simulink model "Telescope_model_MPC"  (R2024b)
settings: Solver=ode4  StartTime=0.0  StopTime=SimulationTime  FixedStep=Tc  RelTol=1e-5
undefined symbols (not defined in the file): APaz, APel, Arcs2Deg, BPaz, BPel, CPaz, CPel, Deg2Arcs, DPaz, DPel, Prepocessor, Scenario, sgn, VonKarman, x0_az, x0_el
libraries: simulink x18, mpclib x1
(part 1 of 2)
settings Model: Creator=giaco  LastModifiedBy=giacomobasile
settings DebuggingCC: UnderSpecifiedDimensionMsg=warning
settings RTWCC: GPUComputeCapability=3.5

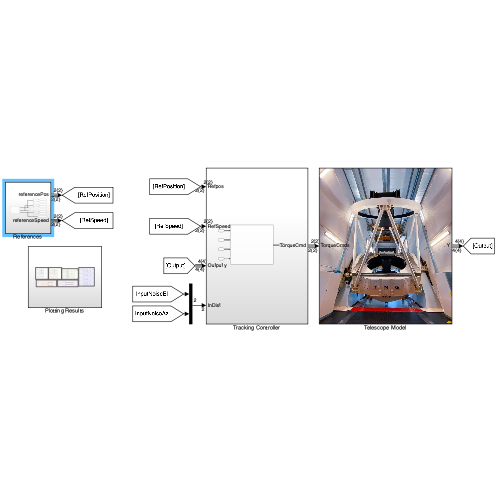
[thumbnail: Simulink's stored preview of the top-level diagram]
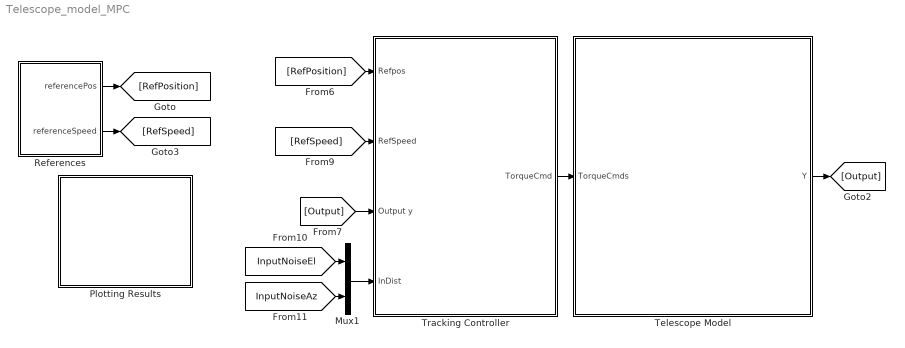
== system Telescope_model_MPC ==
  Mux1 : Mux  Inputs=2
  Plotting Results : Subsystem
  References : Subsystem
  Telescope Model : Subsystem
      mask Display: image('tng1_1.jpg');
  Tracking Controller : Subsystem
  wires:
  [InputNoiseAz] -> Mux1/2
  [RefSpeed] -> Tracking Controller/2(RefSpeed)
  [Output] -> Tracking Controller/3(Output y)
  Mux1/1 -> Tracking Controller/4(InDist)
  [RefPosition] -> Tracking Controller/1(Refpos)
  [InputNoiseEl] -> Mux1/1
  References/2(referenceSpeed) -> [RefSpeed]
  References/1(referencePos) -> [RefPosition]
  Telescope Model/1(Y) -> [Output]
  Tracking Controller/1(TorqueCmd) -> Telescope Model/1(TorqueCmds)

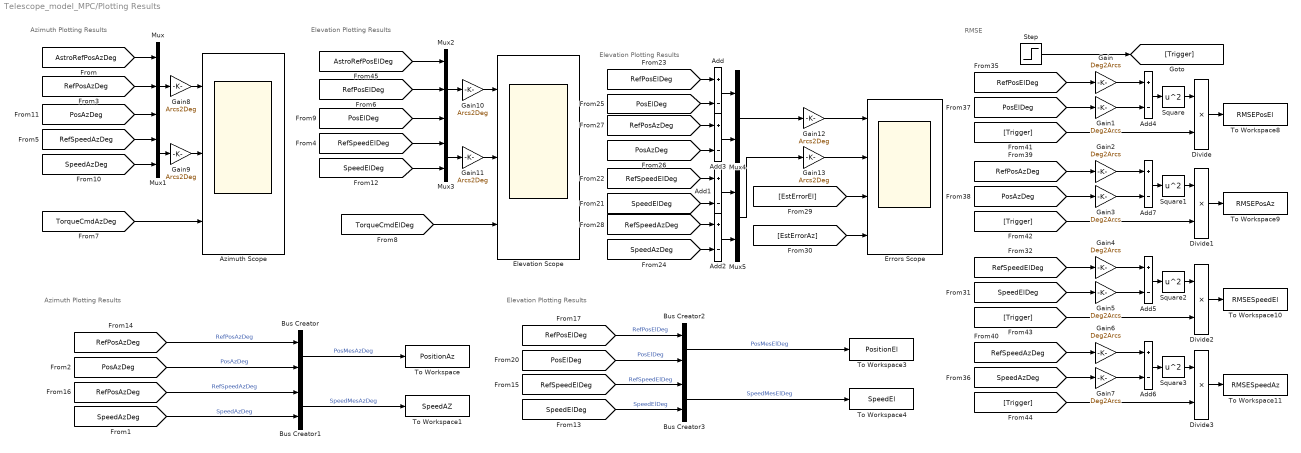
== system Telescope_model_MPC/Plotting Results ==
  note: RMSE
  note: Azimuth Plotting Results
  note: Elevation Plotting Results
  note: Elevation Plotting Results
  note: Azimuth Plotting Results
  note: Elevation Plotting Results
  Add{,1..7} (8 alike) : Sum  Inputs=+-
  Azimuth Scope : Scope  NumInputPorts=3
  Bus Creator{,1..3} (4 alike) : BusCreator  Inputs=2
  Divide{,1..3} (4 alike) : Product  Inputs=**
  Elevation Scope : Scope  NumInputPorts=3
  Errors Scope : Scope  NumInputPorts=4
  Gain{,1..7} (8 alike) : Gain  Gain=Deg2Arcs
  Gain{8..13} (6 alike) : Gain  Gain=Arcs2Deg
  Mux : Mux  Inputs=3
  Mux{1,3..5} (4 alike) : Mux  Inputs=2
  Mux2 : Mux  Inputs=3
  Square{,1..3} (4 alike) : Math  Operator=square
  Step : Step  Time=350  SampleTime=0
  To Workspace : ToWorkspace  VariableName=PositionAz  SaveFormat=Timeseries  SampleTime=-1
  To Workspace1 : ToWorkspace  VariableName=SpeedAZ  SaveFormat=Timeseries  SampleTime=-1
  To Workspace10 : ToWorkspace  VariableName=RMSESpeedEl  SaveFormat=Timeseries  SampleTime=-1
  To Workspace11 : ToWorkspace  VariableName=RMSESpeedAz  SaveFormat=Timeseries  SampleTime=-1
  To Workspace3 : ToWorkspace  VariableName=PositionEl  SaveFormat=Timeseries  SampleTime=-1
  To Workspace4 : ToWorkspace  VariableName=SpeedEl  SaveFormat=Timeseries  SampleTime=-1
  To Workspace8 : ToWorkspace  VariableName=RMSEPosEl  SaveFormat=Timeseries  SampleTime=-1
  To Workspace9 : ToWorkspace  VariableName=RMSEPosAz  SaveFormat=Timeseries  SampleTime=-1
  wires:
  [RefPosAzDeg] -> Mux/2
  [PosAzDeg] -> Mux/3
  [RefSpeedAzDeg] -> Mux1/1
  [SpeedAzDeg] -> Mux1/2
  Mux/1 -> Gain8/1
  Mux1/1 -> Gain9/1
  [TorqueCmdAzDeg] -> Azimuth Scope/3
  [TorqueCmdElDeg] -> Elevation Scope/3
  Mux3/1 -> Gain11/1
  Mux2/1 -> Gain10/1
  [SpeedElDeg] -> Mux3/2
  [RefSpeedElDeg] -> Mux3/1
  [PosElDeg] -> Mux2/3
  [RefPosElDeg] -> Mux2/2
  [PosAzDeg] -> Bus Creator/2  "PosAzDeg"
  [SpeedAzDeg] -> Bus Creator1/2  "SpeedAzDeg"
  [RefPosAzDeg] -> Bus Creator/1  "RefPosAzDeg"
  [RefPosAzDeg] -> Bus Creator1/1  "RefSpeedAzDeg"
  [RefPosElDeg] -> Bus Creator2/1  "RefPosElDeg"
  [PosElDeg] -> Bus Creator2/2  "PosElDeg"
  [RefSpeedElDeg] -> Bus Creator3/1  "RefSpeedElDeg"
  [SpeedElDeg] -> Bus Creator3/2  "SpeedElDeg"
  Bus Creator/1 -> To Workspace/1  "PosMesAzDeg"
  Bus Creator1/1 -> To Workspace1/1  "SpeedMesAzDeg"
  Bus Creator2/1 -> To Workspace3/1  "PosMesElDeg"
  Bus Creator3/1 -> To Workspace4/1  "SpeedMesElDeg"
  [RefPosElDeg] -> Add/1
  [PosElDeg] -> Add/2
  [RefSpeedElDeg] -> Add1/1
  [SpeedElDeg] -> Add1/2
  [RefSpeedAzDeg] -> Add2/1
  [SpeedAzDeg] -> Add2/2
  [RefPosAzDeg] -> Add3/1
  [PosAzDeg] -> Add3/2
  Add/1 -> Mux4/1
  Add3/1 -> Mux4/2
  Add1/1 -> Mux5/1
  Add2/1 -> Mux5/2
  Mux4/1 -> Gain12/1
  Mux5/1 -> Gain13/1
  [EstErrorEl] -> Errors Scope/3
  [EstErrorAz] -> Errors Scope/4
  Add6/1 -> Square3/1
  Add5/1 -> Square2/1
  Add7/1 -> Square1/1
  Add4/1 -> Square/1
  [PosAzDeg] -> Gain3/1
  [RefPosAzDeg] -> Gain2/1
  [SpeedAzDeg] -> Gain7/1
  [RefSpeedAzDeg] -> Gain6/1
  [SpeedElDeg] -> Gain5/1
  [RefSpeedElDeg] -> Gain4/1
  [PosElDeg] -> Gain1/1
  [RefPosElDeg] -> Gain/1
  Square/1 -> Divide/1
  Divide/1 -> To Workspace8/1
  Step/1 -> [Trigger]
  [Trigger] -> Divide/2
  [Trigger] -> Divide1/2
  Square1/1 -> Divide1/1
  Divide1/1 -> To Workspace9/1
  [Trigger] -> Divide2/2
  Square2/1 -> Divide2/1
  Divide2/1 -> To Workspace10/1
  [Trigger] -> Divide3/2
  Square3/1 -> Divide3/1
  Divide3/1 -> To Workspace11/1
  Gain/1 -> Add4/1
  Gain1/1 -> Add4/2
  Gain2/1 -> Add7/1
  Gain3/1 -> Add7/2
  Gain4/1 -> Add5/1
  Gain5/1 -> Add5/2
  Gain6/1 -> Add6/1
  Gain7/1 -> Add6/2
  [AstroRefPosElDeg] -> Mux2/1
  [AstroRefPosAzDeg] -> Mux/1
  Gain8/1 -> Azimuth Scope/1
  Gain9/1 -> Azimuth Scope/2
  Gain10/1 -> Elevation Scope/1
  Gain11/1 -> Elevation Scope/2
  Gain12/1 -> Errors Scope/1
  Gain13/1 -> Errors Scope/2

== system Telescope_model_MPC/References ==
  Bus Selector : BusSelector  OutputSignals=Azimuth,Elevation
  Bus Selector1 : BusSelector  OutputSignals=ElevationPosition,AzimuthPosition
  Bus Selector2 : BusSelector  OutputSignals=Azimuth,Elevation
  References : Subsystem  Variant=on  VariantControl=Choice
  To Workspace : ToWorkspace  VariableName=AstroReference  SaveFormat=Timeseries  SampleTime=-1
  referencePos : Outport
  referenceSpeed : Outport  Port=2
  tag scope: AstroRefPosAzDeg=global, AstroRefPosElDeg=global, RefPosAzDeg=global, RefPosElDeg=global, RefSpeedAzDeg=global, RefSpeedElDeg=global
  wires:
  References/1(referencePos) -> Bus Selector/1, referencePos/1  "[Deg]"
  Bus Selector/1 -> [RefPosAzDeg]  "<Azimuth>"
  Bus Selector/2 -> [RefPosElDeg]  "<Elevation>"
  Bus Selector1/2 -> [AstroRefPosAzDeg]  "<AzimuthPosition>"
  Bus Selector1/1 -> [AstroRefPosElDeg]  "<ElevationPosition>"
  References/3(AstroReference) -> To Workspace/1, Bus Selector1/1  "[Deg]"
  Bus Selector2/2 -> [RefSpeedElDeg]  "<Elevation>"
  Bus Selector2/1 -> [RefSpeedAzDeg]  "<Azimuth>"
  References/2(referenceSpeed) -> Bus Selector2/1, referenceSpeed/1  "[Deg]"

== system Telescope_model_MPC/Telescope Model ==
  note: Input Management Section
  note: Models dynamics
  TorqueCmds : Inport
  Azimuth Model : Subsystem
  Bus Selector : BusSelector  OutputSignals=Elevation,Azimuth
  Demux : Demux  Outputs=2
  Demux1 : Demux  Outputs=2
  Elevation Model : Subsystem
  Scope : Scope  NumInputPorts=2
  To Workspace1 : ToWorkspace  VariableName=TorqueAz  SaveFormat=Timeseries  SampleTime=-1
  To Workspace3 : ToWorkspace  VariableName=TorqueEl  SaveFormat=Timeseries  SampleTime=-1
  Out Bus Element2 : Outport  PortName=Y  Element=ElevationSpeed
  Out Bus Element3 : Outport  PortName=Y  Element=ElevationPosition
  Out Bus Element4 : Outport  PortName=Y  Element=AzimuthSpeed
  Out Bus Element5 : Outport  PortName=Y  Element=AzimuthPosition
  tag scope: PosAzDeg=global, PosElDeg=global, SpeedAzDeg=global, SpeedElDeg=global, TorqueCmdAzDeg=global, TorqueCmdElDeg=global
  wires:
  TorqueCmds/1 -> Bus Selector/1
  Azimuth Model/1(y) -> Demux1/1, Scope/2  "[Arcs]"
  Elevation Model/1(y) -> Scope/1, Demux/1  "[Arcs]"
  Bus Selector/1 -> To Workspace3/1, [TorqueCmdElDeg]  "<Elevation>"
  Bus Selector/2 -> To Workspace1/1, [TorqueCmdAzDeg]  "<Azimuth>"
  [TorqueCmdElDeg] -> Elevation Model/1(Torque)
  [TorqueCmdAzDeg] -> Azimuth Model/1(Troque)
  Demux/2 -> [SpeedElDeg], Out Bus Element2/1
  Demux/1 -> Out Bus Element3/1, [PosElDeg]
  Demux1/1 -> Out Bus Element5/1, [PosAzDeg]
  Demux1/2 -> [SpeedAzDeg], Out Bus Element4/1

== system Telescope_model_MPC/Tracking Controller ==
  Refpos : Inport
  RefSpeed : Inport  Port=2
  Output y : Inport  Port=3
  InDist : Inport  Port=4
  Tracking_Controller_MPC : Subsystem  TreatAsAtomicUnit=on  VariantControl=CtrMode == 3 && NNFConf == 2
  TorqueCmd : Outport
  wires:
  Refpos/1 -> Tracking_Controller_MPC/1(Refpos)
  Output y/1 -> Tracking_Controller_MPC/3(Output y)
  Tracking_Controller_MPC/1(TorqueCmd) -> TorqueCmd/1
  RefSpeed/1 -> Tracking_Controller_MPC/2(RefSpeed)
  InDist/1 -> Tracking_Controller_MPC/4(InDist)

== system Telescope_model_MPC/References/References ==
  " References from TNG" : Subsystem  VariantControl=Ref == 0 && Prepocessor.flag == 0 && TNG==1
  Astrometric Computation : Subsystem  VariantControl=Ref == 0 && Prepocessor.flag == 0 && TNG==0
  Prepocessed Trivial References PID/LQG : Subsystem  VariantControl=Ref == 1
  Preprocessed Astrometric Computation : Subsystem  VariantControl=Ref == 0 && Prepocessor.flag == 1 && TNG==0
  Preprocessed Astrometric References from TNG : Subsystem  VariantControl=Ref == 0 && Prepocessor.flag == 1 && TNG==1
  Trivial References PID/LQG : Subsystem  VariantControl=Ref == 1
  referencePos : Outport
  referenceSpeed : Outport  Port=2
  AstroReference : Outport  Port=3

== system Telescope_model_MPC/Telescope Model/Azimuth Model ==
  Troque : Inport
  Add : Sum
  Add1 : Sum
  Integrator : Integrator  InitialCondition=x0_az
  Noise Model : Subsystem  Variant=on  VariantControl=Choice
  Scope : Scope  NumInputPorts=2
  Sum : Sum  Inputs=++|
  Sum1 : Sum  Inputs=++|
  sys.A : Gain  Gain=APaz  Multiplication=Matrix(K*u)
  sys.B : Gain  Gain=BPaz  Multiplication=Matrix(K*u)
  sys.C : Gain  Gain=CPaz  Multiplication=Matrix(K*u)
  sys.D : Gain  Gain=DPaz  Multiplication=Matrix(K*u)
  y : Outport
  tag scope: InputNoiseAz=global
  wires:
  Add1/1 -> Integrator/1
  sys.C/1 -> Add/2
  sys.D/1 -> Add/1
  Sum1/1 -> sys.B/1, sys.D/1
  Sum/1 -> y/1
  Add/1 -> Sum/2
  Troque/1 -> Sum1/2
  Noise Model/1(d_out) -> Scope/1, Sum/1
  sys.B/1 -> Add1/1
  sys.A/1 -> Add1/2
  Integrator/1 -> sys.A/1, sys.C/1
  Noise Model/2(d_in) -> [InputNoiseAz], Sum1/1, Scope/2

== system Telescope_model_MPC/Telescope Model/Elevation Model ==
  Torque : Inport
  Add : Sum
  Add1 : Sum
  Integrator : Integrator  InitialCondition=x0_el
  Noise Model : Subsystem  Variant=on  VariantControl=Choice
  Scope : Scope  NumInputPorts=2
  Sum : Sum  Inputs=++|
  Sum1 : Sum  Inputs=++|
  sys.A : Gain  Gain=APel  Multiplication=Matrix(K*u)
  sys.B : Gain  Gain=BPel  Multiplication=Matrix(K*u)
  sys.C : Gain  Gain=CPel  Multiplication=Matrix(K*u)
  sys.D : Gain  Gain=DPel  Multiplication=Matrix(K*u)
  y : Outport
  tag scope: InputNoiseEl=global
  wires:
  sys.B/1 -> Add1/1
  sys.C/1 -> Add/2
  sys.D/1 -> Add/1
  Add/1 -> Sum/2
  Sum/1 -> y/1
  Sum1/1 -> sys.B/1, sys.D/1
  Torque/1 -> Sum1/2
  Noise Model/1(d_out) -> Scope/1, Sum/1
  Noise Model/2(d_in) -> [InputNoiseEl], Sum1/1, Scope/2
  sys.A/1 -> Add1/2
  Add1/1 -> Integrator/1
  Integrator/1 -> sys.A/1, sys.C/1

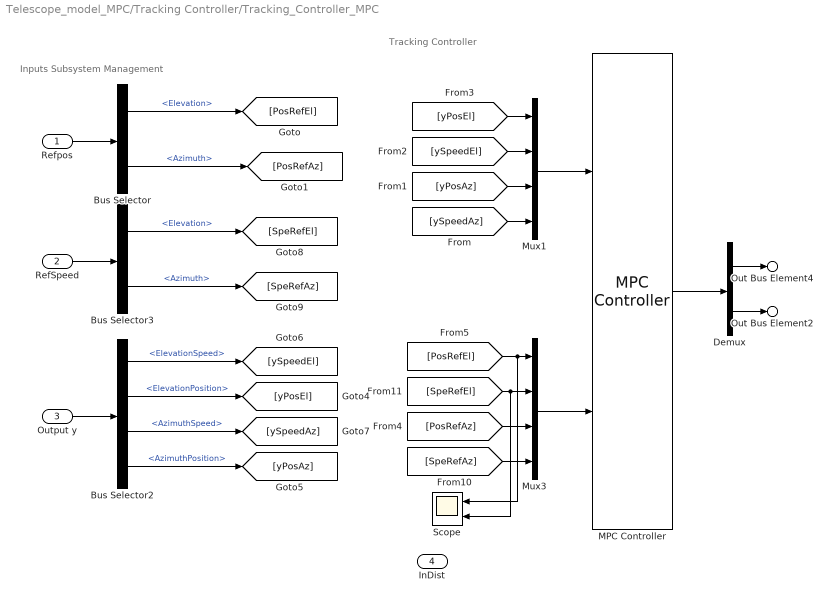
== system Telescope_model_MPC/Tracking Controller/Tracking_Controller_MPC ==
  note: Inputs Subsystem Management
  note: Tracking Controller
  Refpos : Inport
  RefSpeed : Inport  Port=2
  Output y : Inport  Port=3
  InDist : Inport  Port=4
  Bus Selector : BusSelector  OutputSignals=Elevation,Azimuth
  Bus Selector2 : BusSelector  OutputSignals=ElevationSpeed,ElevationPosition,AzimuthSpeed,AzimuthPosition
  Bus Selector3 : BusSelector  OutputSignals=Elevation,Azimuth
  Demux : Demux  Outputs=2
  MPC Controller : mpclib/MPC Controller  SCDEnableBlockLinearizationSpecification=on  mpcobj=mpcobj  is_multiple=0  enable_value=0  return_u0=off  updateMPCinCallerWorkspace=on  md_inport=off  mv_inport=off  uref_inport=off  return_cost=off  return_mvseq=off  return_qpstatus=off  return_xseq=off  return_state=off  return_ovseq=off  state_inport=off  umin_inport=off  umax_inport=off  ymin_inport=off  ymax_inport=off  cc_inport=off  ywt_inport=off  uwt_inport=off  duwt_inport=off  rhoeps_inport=off  pm_inport=off  MaximumP=10  HorizonChoice=FixedHorizon  n_ts=0.002  n_p=1000  n_mv=2  n_md=0  n_ud=0  n_mo=4  n_uo=0  BlockDataType=double  SampleTimeInherited=off  switch_inport=off
  Mux1 : Mux
  Mux3 : Mux
  Scope : Scope  NumInputPorts=2
  Out Bus Element2 : Outport  PortName=TorqueCmd  Element=Azimuth
  Out Bus Element4 : Outport  PortName=TorqueCmd  Element=Elevation
  wires:
  Bus Selector2/2 -> [yPosEl]  "<ElevationPosition>"
  Bus Selector2/1 -> [ySpeedEl]  "<ElevationSpeed>"
  Bus Selector2/3 -> [ySpeedAz]  "<AzimuthSpeed>"
  Bus Selector2/4 -> [yPosAz]  "<AzimuthPosition>"
  Output y/1 -> Bus Selector2/1
  Bus Selector/2 -> [PosRefAz]  "<Azimuth>"
  Bus Selector/1 -> [PosRefEl]  "<Elevation>"
  Refpos/1 -> Bus Selector/1
  MPC Controller/1 -> Demux/1
  Bus Selector3/1 -> [SpeRefEl]  "<Elevation>"
  Bus Selector3/2 -> [SpeRefAz]  "<Azimuth>"
  RefSpeed/1 -> Bus Selector3/1
  Mux3/1 -> MPC Controller/2
  Mux1/1 -> MPC Controller/1
  [PosRefAz] -> Mux3/3
  [SpeRefAz] -> Mux3/4
  [yPosAz] -> Mux1/3
  [ySpeedAz] -> Mux1/4
  [SpeRefEl] -> Scope/2, Mux3/2
  [PosRefEl] -> Scope/1, Mux3/1
  [yPosEl] -> Mux1/1
  [ySpeedEl] -> Mux1/2
  Demux/1 -> Out Bus Element4/1
  Demux/2 -> Out Bus Element2/1

== system Telescope_model_MPC/References/References/ References from TNG ==
  Discrete Derivative : simulink/Discrete/Discrete Derivative  gainval=1.0  ICPrevScaledInput=0.0  OutMin=[]  OutMax=[]  OutDataType=fixdt(1, 16)  OutScaling=2^-10  DoSatur=off
  Discrete Derivative1 : simulink/Discrete/Discrete Derivative  gainval=1.0  ICPrevScaledInput=0.0  OutMin=[]  OutMax=[]  OutDataType=fixdt(1, 16)  OutScaling=2^-10  DoSatur=off
  From Workspace : FromWorkspace  VariableName=Scenario.AzimuthPosition
  From Workspace1 : FromWorkspace  VariableName=Scenario.ElevationPosition
  Out Bus Element : Outport  PortName=referencePos  Element=Azimuth
  Out Bus Element1 : Outport  PortName=referencePos  Element=Elevation
  Out Bus Element2 : Outport  Port=2  PortName=referenceSpeed  Element=Azimuth
  Out Bus Element3 : Outport  Port=2  PortName=referenceSpeed  Element=Elevation
  Out Bus Element4 : Outport  Port=3  PortName=AstroReference  Element=AzimuthSpeed
  Out Bus Element5 : Outport  Port=3  PortName=AstroReference  Element=ElevationPosition
  Out Bus Element6 : Outport  Port=3  PortName=AstroReference  Element=AzimuthPosition
  Out Bus Element7 : Outport  Port=3  PortName=AstroReference  Element=ElevationSpeed
  wires:
  From Workspace/1 -> Discrete Derivative1/1, Out Bus Element6/1, Out Bus Element/1  "[Arcs]"
  From Workspace1/1 -> Discrete Derivative/1, Out Bus Element5/1, Out Bus Element1/1  "[Arcs]"
  Discrete Derivative1/1 -> Out Bus Element4/1, Out Bus Element2/1
  Discrete Derivative/1 -> Out Bus Element7/1, Out Bus Element3/1

== system Telescope_model_MPC/References/References/Astrometric Computation ==
  Clock : Clock
  Constant10 : Constant  Value=Scenario.VLT
  Constant11 : Constant  Value=Scenario.Time
  Constant19 : Constant  Value=Scenario.RAhh
  Constant21 : Constant  Value=Scenario.DECdd
  Constant3 : Constant  Value=Scenario.RAmm
  Constant4 : Constant  Value=Scenario.RAss
  Constant6 : Constant  Value=Scenario.DECmm
  Constant7 : Constant  Value=Scenario.DECss
  Constant8 : Constant  Value=Scenario.LATsite
  Constant9 : Constant  Value=Scenario.LONsite
  Discrete Derivative{,1..3} (4 alike) : simulink/Discrete/Discrete Derivative  gainval=1.0  ICPrevScaledInput=0.0  OutMin=[]  OutMax=[]  OutDataType=fixdt(1, 16)  OutScaling=2^-10  DoSatur=off
  MATLAB Function : MATLAB Function  TreatAsAtomicUnit=on
  Scope2 : Scope
  Out Bus Element : Outport  PortName=referencePos  Element=Azimuth
  Out Bus Element1 : Outport  PortName=referencePos  Element=Elevation
  Out Bus Element2 : Outport  Port=2  PortName=referenceSpeed  Element=Azimuth
  Out Bus Element3 : Outport  Port=2  PortName=referenceSpeed  Element=Elevation
  Out Bus Element4 : Outport  Port=3  PortName=AstroReference  Element=AzimuthSpeed
  Out Bus Element5 : Outport  Port=3  PortName=AstroReference  Element=ElevationPosition
  Out Bus Element6 : Outport  Port=3  PortName=AstroReference  Element=AzimuthPosition
  Out Bus Element7 : Outport  Port=3  PortName=AstroReference  Element=ElevationSpeed
  wires:
  Discrete Derivative1/1 -> Out Bus Element7/1
  Constant9/1 -> MATLAB Function/10(Longitude)
  Constant19/1 -> MATLAB Function/3(RAhh)
  Constant3/1 -> MATLAB Function/4(RAmm)
  Constant21/1 -> MATLAB Function/6(DECdd)
  Clock/1 -> Scope2/1, MATLAB Function/1(clo)
  Discrete Derivative3/1 -> Out Bus Element3/1
  Constant4/1 -> MATLAB Function/5(RAss)
  Constant7/1 -> MATLAB Function/8(DECss)
  Constant6/1 -> MATLAB Function/7(DECmm)
  Constant10/1 -> MATLAB Function/11(VLT)
  Constant11/1 -> MATLAB Function/2(Time)
  Discrete Derivative2/1 -> Out Bus Element2/1
  Constant8/1 -> MATLAB Function/9(Latitude)
  MATLAB Function/1(Az) -> Discrete Derivative/1, Out Bus Element6/1, Discrete Derivative2/1, Out Bus Element/1
  MATLAB Function/2(Alt) -> Discrete Derivative3/1, Out Bus Element5/1, Discrete Derivative1/1, Out Bus Element1/1
  Discrete Derivative/1 -> Out Bus Element4/1

== system Telescope_model_MPC/References/References/Prepocessed Trivial References PID//LQG ==
  Add1 : Sum  Inputs=+-
  Add2 : Sum  Inputs=+-
  Discrete Derivative : simulink/Discrete/Discrete Derivative  gainval=1.0  ICPrevScaledInput=0.0  OutMin=[]  OutMax=[]  OutDataType=fixdt(1, 16)  OutScaling=2^-10  DoSatur=off
  Discrete Derivative1 : simulink/Discrete/Discrete Derivative  gainval=1.0  ICPrevScaledInput=0.0  OutMin=[]  OutMax=[]  OutDataType=fixdt(1, 16)  OutScaling=2^-10  DoSatur=off
  Gain{6..13} (8 alike) : Gain  Gain=Deg2Arcs
  Integrator1 : Integrator
  Integrator2 : Integrator
  Prepocessor Azimuth : Subsystem
  Prepocessor Elavation : Subsystem
  Step1 : Step  Time=2  After=5  SampleTime=0
  Step2 : Step  Time=12  After=5  SampleTime=0
  Step4 : Step  Time=20  After=0.2  SampleTime=0
  Step5 : Step  Time=30  After=0.2  SampleTime=0
  Out Bus Element : Outport  PortName=referencePos  Element=Azimuth
  Out Bus Element1 : Outport  PortName=referencePos  Element=Elevation
  Out Bus Element2 : Outport  Port=2  PortName=referenceSpeed  Element=Azimuth
  Out Bus Element3 : Outport  Port=2  PortName=referenceSpeed  Element=Elevation
  Out Bus Element4 : Outport  Port=3  PortName=AstroReference  Element=AzimuthSpeed
  Out Bus Element5 : Outport  Port=3  PortName=AstroReference  Element=ElevationPosition
  Out Bus Element6 : Outport  Port=3  PortName=AstroReference  Element=AzimuthPosition
  Out Bus Element7 : Outport  Port=3  PortName=AstroReference  Element=ElevationSpeed
  wires:
  Step4/1 -> Add2/1
  Step5/1 -> Add2/2
  Step2/1 -> Add1/2
  Step1/1 -> Add1/1
  Add1/1 -> Integrator1/1  "[Deg]"
  Add2/1 -> Integrator2/1  "[Deg]"
  Gain6/1 -> Out Bus Element/1
  Gain11/1 -> Out Bus Element5/1
  Gain10/1 -> Out Bus Element7/1
  Gain7/1 -> Out Bus Element2/1
  Gain13/1 -> Out Bus Element3/1
  Gain9/1 -> Out Bus Element4/1
  Prepocessor Azimuth/2(ReferenceSpeed) -> Gain7/1
  Prepocessor Azimuth/1(ReferencePosition) -> Gain6/1
  Prepocessor Elavation/1(ReferencePosition) -> Gain12/1
  Prepocessor Elavation/2(ReferenceSpeed) -> Gain13/1
  Gain8/1 -> Out Bus Element6/1
  Integrator1/1 -> Discrete Derivative1/1, Gain8/1, Prepocessor Azimuth/1(Astrometry Computation)  "[Deg]"
  Integrator2/1 -> Prepocessor Elavation/1(Astrometry Computation), Discrete Derivative/1, Gain11/1  "[Deg]"
  Gain12/1 -> Out Bus Element1/1
  Discrete Derivative1/1 -> Gain9/1
  Discrete Derivative/1 -> Gain10/1

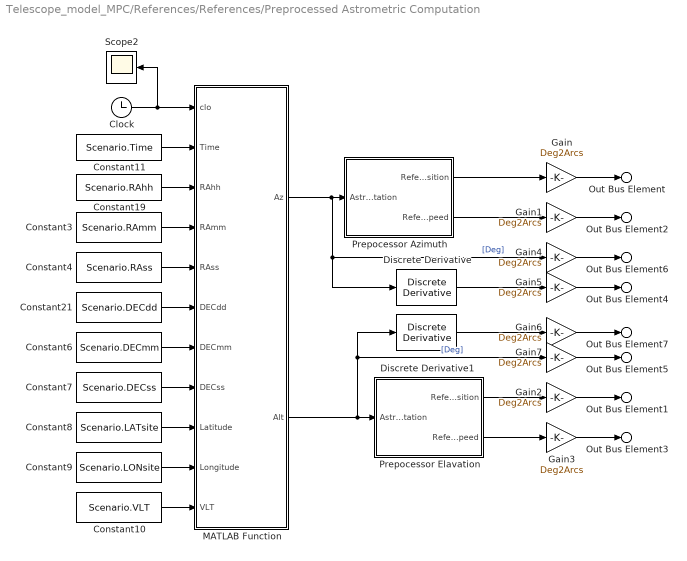
== system Telescope_model_MPC/References/References/Preprocessed Astrometric Computation ==
  Clock : Clock
  Constant10 : Constant  Value=Scenario.VLT
  Constant11 : Constant  Value=Scenario.Time
  Constant19 : Constant  Value=Scenario.RAhh
  Constant21 : Constant  Value=Scenario.DECdd
  Constant3 : Constant  Value=Scenario.RAmm
  Constant4 : Constant  Value=Scenario.RAss
  Constant6 : Constant  Value=Scenario.DECmm
  Constant7 : Constant  Value=Scenario.DECss
  Constant8 : Constant  Value=Scenario.LATsite
  Constant9 : Constant  Value=Scenario.LONsite
  Discrete Derivative : simulink/Discrete/Discrete Derivative  gainval=1.0  ICPrevScaledInput=0.0  OutMin=[]  OutMax=[]  OutDataType=fixdt(1, 16)  OutScaling=2^-10  DoSatur=off
  Discrete Derivative1 : simulink/Discrete/Discrete Derivative  gainval=1.0  ICPrevScaledInput=0.0  OutMin=[]  OutMax=[]  OutDataType=fixdt(1, 16)  OutScaling=2^-10  DoSatur=off
  Gain{,1..7} (8 alike) : Gain  Gain=Deg2Arcs
  MATLAB Function : MATLAB Function  TreatAsAtomicUnit=on
  Prepocessor Azimuth : Subsystem
  Prepocessor Elavation : Subsystem
  Scope2 : Scope
  Out Bus Element : Outport  PortName=referencePos  Element=Azimuth
  Out Bus Element1 : Outport  PortName=referencePos  Element=Elevation
  Out Bus Element2 : Outport  Port=2  PortName=referenceSpeed  Element=Azimuth
  Out Bus Element3 : Outport  Port=2  PortName=referenceSpeed  Element=Elevation
  Out Bus Element4 : Outport  Port=3  PortName=AstroReference  Element=AzimuthSpeed
  Out Bus Element5 : Outport  Port=3  PortName=AstroReference  Element=ElevationPosition
  Out Bus Element6 : Outport  Port=3  PortName=AstroReference  Element=AzimuthPosition
  Out Bus Element7 : Outport  Port=3  PortName=AstroReference  Element=ElevationSpeed
  wires:
  Constant21/1 -> MATLAB Function/6(DECdd)
  Constant7/1 -> MATLAB Function/8(DECss)
  Constant11/1 -> MATLAB Function/2(Time)
  Constant6/1 -> MATLAB Function/7(DECmm)
  Constant10/1 -> MATLAB Function/11(VLT)
  Clock/1 -> Scope2/1, MATLAB Function/1(clo)
  Constant4/1 -> MATLAB Function/5(RAss)
  Constant8/1 -> MATLAB Function/9(Latitude)
  Constant3/1 -> MATLAB Function/4(RAmm)
  Constant9/1 -> MATLAB Function/10(Longitude)
  Constant19/1 -> MATLAB Function/3(RAhh)
  MATLAB Function/1(Az) -> Gain4/1, Discrete Derivative/1, Prepocessor Azimuth/1(Astrometry Computation)  "[Deg]"
  MATLAB Function/2(Alt) -> Discrete Derivative1/1, Gain7/1, Prepocessor Elavation/1(Astrometry Computation)  "[Deg]"
  Prepocessor Azimuth/2(ReferenceSpeed) -> Gain1/1
  Prepocessor Azimuth/1(ReferencePosition) -> Gain/1
  Prepocessor Elavation/2(ReferenceSpeed) -> Gain3/1
  Prepocessor Elavation/1(ReferencePosition) -> Gain2/1
  Discrete Derivative/1 -> Gain5/1
  Discrete Derivative1/1 -> Gain6/1
  Gain/1 -> Out Bus Element/1
  Gain1/1 -> Out Bus Element2/1
  Gain2/1 -> Out Bus Element1/1
  Gain3/1 -> Out Bus Element3/1
  Gain4/1 -> Out Bus Element6/1
  Gain5/1 -> Out Bus Element4/1
  Gain6/1 -> Out Bus Element7/1
  Gain7/1 -> Out Bus Element5/1

== system Telescope_model_MPC/References/References/Preprocessed Astrometric References from TNG ==
  Discrete Derivative : simulink/Discrete/Discrete Derivative  gainval=1.0  ICPrevScaledInput=0.0  OutMin=[]  OutMax=[]  OutDataType=fixdt(1, 16)  OutScaling=2^-10  DoSatur=off
  Discrete Derivative1 : simulink/Discrete/Discrete Derivative  gainval=1.0  ICPrevScaledInput=0.0  OutMin=[]  OutMax=[]  OutDataType=fixdt(1, 16)  OutScaling=2^-10  DoSatur=off
  From Workspace : FromWorkspace  VariableName=Scenario.AzimuthPosition
  From Workspace1 : FromWorkspace  VariableName=Scenario.ElevationPosition
  Gain : Gain  Gain=Arcs2Deg
  Gain1 : Gain  Gain=Arcs2Deg
  Gain{2..9} (8 alike) : Gain  Gain=Deg2Arcs
  Prepocessor Azimuth : Subsystem
  Prepocessor Elavation : Subsystem
  Out Bus Element : Outport  PortName=referencePos  Element=Azimuth
  Out Bus Element1 : Outport  PortName=referencePos  Element=Elevation
  Out Bus Element2 : Outport  Port=2  PortName=referenceSpeed  Element=Azimuth
  Out Bus Element3 : Outport  Port=2  PortName=referenceSpeed  Element=Elevation
  Out Bus Element4 : Outport  Port=3  PortName=AstroReference  Element=AzimuthSpeed
  Out Bus Element5 : Outport  Port=3  PortName=AstroReference  Element=ElevationPosition
  Out Bus Element6 : Outport  Port=3  PortName=AstroReference  Element=AzimuthPosition
  Out Bus Element7 : Outport  Port=3  PortName=AstroReference  Element=ElevationSpeed
  wires:
  Discrete Derivative/1 -> Gain6/1
  Discrete Derivative1/1 -> Gain5/1
  Prepocessor Elavation/1(ReferencePosition) -> Gain8/1
  Prepocessor Elavation/2(ReferenceSpeed) -> Gain9/1
  Prepocessor Azimuth/1(ReferencePosition) -> Gain2/1
  Prepocessor Azimuth/2(ReferenceSpeed) -> Gain3/1
  From Workspace/1 -> Gain/1  "[Arcs]"
  Gain/1 -> Prepocessor Azimuth/1(Astrometry Computation), Discrete Derivative1/1, Gain4/1  "[Deg]"
  Gain1/1 -> Prepocessor Elavation/1(Astrometry Computation), Discrete Derivative/1, Gain7/1  "[Deg]"
  From Workspace1/1 -> Gain1/1  "[Arcs]"
  Gain2/1 -> Out Bus Element/1
  Gain3/1 -> Out Bus Element2/1
  Gain4/1 -> Out Bus Element6/1
  Gain5/1 -> Out Bus Element4/1
  Gain6/1 -> Out Bus Element7/1
  Gain7/1 -> Out Bus Element5/1
  Gain8/1 -> Out Bus Element1/1
  Gain9/1 -> Out Bus Element3/1

== system Telescope_model_MPC/References/References/Trivial References PID//LQG ==
  Add1 : Sum  Inputs=+-
  Add2 : Sum  Inputs=+-
  Discrete Derivative : simulink/Discrete/Discrete Derivative  gainval=1.0  ICPrevScaledInput=0.0  OutMin=[]  OutMax=[]  OutDataType=fixdt(1, 16)  OutScaling=2^-10  DoSatur=off
  Discrete Derivative1 : simulink/Discrete/Discrete Derivative  gainval=1.0  ICPrevScaledInput=0.0  OutMin=[]  OutMax=[]  OutDataType=fixdt(1, 16)  OutScaling=2^-10  DoSatur=off
  Gain{6..13} (8 alike) : Gain  Gain=Deg2Arcs
  Integrator1 : Integrator
  Integrator2 : Integrator
  Prepocessor Azimuth : Subsystem
  Prepocessor Elavation : Subsystem
  Step1 : Step  Time=2  After=5  SampleTime=0
  Step2 : Step  Time=12  After=5  SampleTime=0
  Step4 : Step  Time=20  After=0.2  SampleTime=0
  Step5 : Step  Time=30  After=0.2  SampleTime=0
  Out Bus Element : Outport  PortName=referencePos  Element=Azimuth
  Out Bus Element1 : Outport  PortName=referencePos  Element=Elevation
  Out Bus Element2 : Outport  Port=2  PortName=referenceSpeed  Element=Azimuth
  Out Bus Element3 : Outport  Port=2  PortName=referenceSpeed  Element=Elevation
  Out Bus Element4 : Outport  Port=3  PortName=AstroReference  Element=AzimuthSpeed
  Out Bus Element5 : Outport  Port=3  PortName=AstroReference  Element=ElevationPosition
  Out Bus Element6 : Outport  Port=3  PortName=AstroReference  Element=AzimuthPosition
  Out Bus Element7 : Outport  Port=3  PortName=AstroReference  Element=ElevationSpeed
  wires:
  Step4/1 -> Add2/1
  Step5/1 -> Add2/2
  Step2/1 -> Add1/2
  Step1/1 -> Add1/1
  Add1/1 -> Integrator1/1  "[Deg]"
  Add2/1 -> Integrator2/1  "[Deg]"
  Gain6/1 -> Out Bus Element/1
  Gain11/1 -> Out Bus Element5/1
  Gain10/1 -> Out Bus Element7/1
  Gain7/1 -> Out Bus Element2/1
  Gain13/1 -> Out Bus Element3/1
  Gain9/1 -> Out Bus Element4/1
  Prepocessor Azimuth/2(ReferenceSpeed) -> Gain7/1
  Prepocessor Azimuth/1(ReferencePosition) -> Gain6/1
  Prepocessor Elavation/1(ReferencePosition) -> Gain12/1
  Prepocessor Elavation/2(ReferenceSpeed) -> Gain13/1
  Gain8/1 -> Out Bus Element6/1
  Integrator1/1 -> Discrete Derivative1/1, Gain8/1, Prepocessor Azimuth/1(Astrometry Computation)  "[Deg]"
  Integrator2/1 -> Prepocessor Elavation/1(Astrometry Computation), Discrete Derivative/1, Gain11/1  "[Deg]"
  Gain12/1 -> Out Bus Element1/1
  Discrete Derivative1/1 -> Gain9/1
  Discrete Derivative/1 -> Gain10/1

== system Telescope_model_MPC/Telescope Model/Azimuth Model/Noise Model ==
  None Noise : Subsystem  VariantControl="NNFConf  == 0"
  Von Karman Torque PSD : Subsystem  VariantControl=NNFConf == 2
  White Noise Output : Subsystem  VariantControl=NNFConf == 1
  d_out : Outport
  d_in : Outport  Port=2

== system Telescope_model_MPC/Telescope Model/Elevation Model/Noise Model ==
  None Noise : Subsystem  VariantControl="NNFConf  == 0"
  Von Karman Torque PSD : Subsystem  VariantControl=NNFConf == 2
  White Noise Output : Subsystem  VariantControl=NNFConf == 1
  d_out : Outport
  d_in : Outport  Port=2

== system Telescope_model_MPC/References/References/Prepocessed Trivial References PID//LQG/Prepocessor Azimuth ==
  Astrometry Computation : Inport
  Integrator : Integrator  InitialCondition=Prepocessor.p0az
  Prepocessor Elevation : Subsystem  TreatAsAtomicUnit=on  SystemSampleTime=Prepocessor.Ts
  Terminator : Terminator
  Terminator1 : Terminator
  To Workspace : ToWorkspace  VariableName=ReferenceProcessedPositionAz  SaveFormat=Timeseries  SampleTime=-1
  To Workspace1 : ToWorkspace  VariableName=ReferenceProcessedSpeedAz  SaveFormat=Timeseries  SampleTime=-1
  Transfer Fcn2 : TransferFcn  Numerator=2500  Denominator=conv([1 50], [1 50])
  ReferencePosition : Outport
  ReferenceSpeed : Outport  Port=2
  wires:
  Prepocessor Elevation/2(speed) -> Transfer Fcn2/1
  Prepocessor Elevation/1(deltaP) -> Terminator/1
  Integrator/1 -> To Workspace/1, ReferencePosition/1
  Prepocessor Elevation/3(PositionRef) -> Terminator1/1
  Transfer Fcn2/1 -> To Workspace1/1, ReferenceSpeed/1, Integrator/1
  Astrometry Computation/1 -> Prepocessor Elevation/1(Az)

== system Telescope_model_MPC/References/References/Prepocessed Trivial References PID//LQG/Prepocessor Elavation ==
  Astrometry Computation : Inport
  Integrator : Integrator  InitialCondition=Prepocessor.p0el
  Prepocessor Elevation : Subsystem  TreatAsAtomicUnit=on  SystemSampleTime=Prepocessor.Ts
  Terminator : Terminator
  Terminator1 : Terminator
  To Workspace : ToWorkspace  VariableName=ReferenceProcessedPositionEl  SaveFormat=Timeseries  SampleTime=-1
  To Workspace1 : ToWorkspace  VariableName=ReferenceProcessedSpeedEl  SaveFormat=Timeseries  SampleTime=-1
  Transfer Fcn2 : TransferFcn  Numerator=2500  Denominator=conv([1 50], [1 50])
  ReferencePosition : Outport
  ReferenceSpeed : Outport  Port=2
  wires:
  Transfer Fcn2/1 -> Integrator/1, To Workspace1/1, ReferenceSpeed/1
  Prepocessor Elevation/3(PositionRef) -> Terminator1/1
  Integrator/1 -> To Workspace/1, ReferencePosition/1
  Prepocessor Elevation/1(deltaP) -> Terminator/1
  Prepocessor Elevation/2(speed) -> Transfer Fcn2/1
  Astrometry Computation/1 -> Prepocessor Elevation/1(El)

== system Telescope_model_MPC/References/References/Preprocessed Astrometric Computation/Prepocessor Azimuth ==
  Astrometry Computation : Inport
  Integrator : Integrator  InitialCondition=Prepocessor.p0az
  Prepocessor Elevation : Subsystem  TreatAsAtomicUnit=on  SystemSampleTime=Prepocessor.Ts
  Terminator : Terminator
  Terminator1 : Terminator
  To Workspace : ToWorkspace  VariableName=ReferenceProcessedPositionAz  SaveFormat=Timeseries  SampleTime=-1
  To Workspace1 : ToWorkspace  VariableName=ReferenceProcessedSpeedAz  SaveFormat=Timeseries  SampleTime=-1
  Transfer Fcn2 : TransferFcn  Numerator=2500  Denominator=conv([1 50], [1 50])
  ReferencePosition : Outport
  ReferenceSpeed : Outport  Port=2
  wires:
  Prepocessor Elevation/2(speed) -> Transfer Fcn2/1
  Prepocessor Elevation/1(deltaP) -> Terminator/1
  Integrator/1 -> To Workspace/1, ReferencePosition/1
  Prepocessor Elevation/3(PositionRef) -> Terminator1/1
  Transfer Fcn2/1 -> To Workspace1/1, ReferenceSpeed/1, Integrator/1
  Astrometry Computation/1 -> Prepocessor Elevation/1(Az)

== system Telescope_model_MPC/References/References/Preprocessed Astrometric Computation/Prepocessor Elavation ==
  Astrometry Computation : Inport
  Integrator : Integrator  InitialCondition=Prepocessor.p0el
  Prepocessor Elevation : Subsystem  TreatAsAtomicUnit=on  SystemSampleTime=Prepocessor.Ts
  Terminator : Terminator
  Terminator1 : Terminator
  To Workspace : ToWorkspace  VariableName=ReferenceProcessedPositionEl  SaveFormat=Timeseries  SampleTime=-1
  To Workspace1 : ToWorkspace  VariableName=ReferenceProcessedSpeedEl  SaveFormat=Timeseries  SampleTime=-1
  Transfer Fcn2 : TransferFcn  Numerator=2500  Denominator=conv([1 50], [1 50])
  ReferencePosition : Outport
  ReferenceSpeed : Outport  Port=2
  wires:
  Transfer Fcn2/1 -> Integrator/1, To Workspace1/1, ReferenceSpeed/1
  Prepocessor Elevation/3(PositionRef) -> Terminator1/1
  Integrator/1 -> To Workspace/1, ReferencePosition/1
  Prepocessor Elevation/1(deltaP) -> Terminator/1
  Prepocessor Elevation/2(speed) -> Transfer Fcn2/1
  Astrometry Computation/1 -> Prepocessor Elevation/1(El)

== system Telescope_model_MPC/References/References/Preprocessed Astrometric References from TNG/Prepocessor Azimuth ==
  Astrometry Computation : Inport
  Integrator : Integrator  InitialCondition=Prepocessor.p0az
  Prepocessor Elevation : Subsystem  TreatAsAtomicUnit=on  SystemSampleTime=Prepocessor.Ts
  Terminator : Terminator
  Terminator1 : Terminator
  To Workspace : ToWorkspace  VariableName=ReferenceProcessedPositionAz  SaveFormat=Timeseries  SampleTime=-1
  To Workspace1 : ToWorkspace  VariableName=ReferenceProcessedSpeedAz  SaveFormat=Timeseries  SampleTime=-1
  Transfer Fcn2 : TransferFcn  Numerator=2500  Denominator=conv([1 50], [1 50])
  ReferencePosition : Outport
  ReferenceSpeed : Outport  Port=2
  wires:
  Prepocessor Elevation/2(speed) -> Transfer Fcn2/1
  Prepocessor Elevation/1(deltaP) -> Terminator/1
  Integrator/1 -> To Workspace/1, ReferencePosition/1
  Prepocessor Elevation/3(PositionRef) -> Terminator1/1
  Transfer Fcn2/1 -> To Workspace1/1, ReferenceSpeed/1, Integrator/1
  Astrometry Computation/1 -> Prepocessor Elevation/1(Az)

== system Telescope_model_MPC/References/References/Preprocessed Astrometric References from TNG/Prepocessor Elavation ==
  Astrometry Computation : Inport
  Integrator : Integrator  InitialCondition=Prepocessor.p0el
  Prepocessor Elevation : Subsystem  TreatAsAtomicUnit=on  SystemSampleTime=Prepocessor.Ts
  Terminator : Terminator
  Terminator1 : Terminator
  To Workspace : ToWorkspace  VariableName=ReferenceProcessedPositionEl  SaveFormat=Timeseries  SampleTime=-1
  To Workspace1 : ToWorkspace  VariableName=ReferenceProcessedSpeedEl  SaveFormat=Timeseries  SampleTime=-1
  Transfer Fcn2 : TransferFcn  Numerator=2500  Denominator=conv([1 50], [1 50])
  ReferencePosition : Outport
  ReferenceSpeed : Outport  Port=2
  wires:
  Transfer Fcn2/1 -> Integrator/1, To Workspace1/1, ReferenceSpeed/1
  Prepocessor Elevation/3(PositionRef) -> Terminator1/1
  Integrator/1 -> To Workspace/1, ReferencePosition/1
  Prepocessor Elevation/1(deltaP) -> Terminator/1
  Prepocessor Elevation/2(speed) -> Transfer Fcn2/1
  Astrometry Computation/1 -> Prepocessor Elevation/1(El)

== system Telescope_model_MPC/References/References/Trivial References PID//LQG/Prepocessor Azimuth ==
  Astrometry Computation : Inport
  Integrator : Integrator  InitialCondition=Prepocessor.p0az
  Prepocessor Elevation : Subsystem  TreatAsAtomicUnit=on  SystemSampleTime=Prepocessor.Ts
  Terminator : Terminator
  Terminator1 : Terminator
  To Workspace : ToWorkspace  VariableName=ReferenceProcessedPositionAz  SaveFormat=Timeseries  SampleTime=-1
  To Workspace1 : ToWorkspace  VariableName=ReferenceProcessedSpeedAz  SaveFormat=Timeseries  SampleTime=-1
  Transfer Fcn2 : TransferFcn  Numerator=2500  Denominator=conv([1 50], [1 50])
  ReferencePosition : Outport
  ReferenceSpeed : Outport  Port=2
  wires:
  Prepocessor Elevation/2(speed) -> Transfer Fcn2/1
  Prepocessor Elevation/1(deltaP) -> Terminator/1
  Integrator/1 -> To Workspace/1, ReferencePosition/1
  Prepocessor Elevation/3(PositionRef) -> Terminator1/1
  Transfer Fcn2/1 -> To Workspace1/1, ReferenceSpeed/1, Integrator/1
  Astrometry Computation/1 -> Prepocessor Elevation/1(Az)

== system Telescope_model_MPC/References/References/Trivial References PID//LQG/Prepocessor Elavation ==
  Astrometry Computation : Inport
  Integrator : Integrator  InitialCondition=Prepocessor.p0el
  Prepocessor Elevation : Subsystem  TreatAsAtomicUnit=on  SystemSampleTime=Prepocessor.Ts
  Terminator : Terminator
  Terminator1 : Terminator
  To Workspace : ToWorkspace  VariableName=ReferenceProcessedPositionEl  SaveFormat=Timeseries  SampleTime=-1
  To Workspace1 : ToWorkspace  VariableName=ReferenceProcessedSpeedEl  SaveFormat=Timeseries  SampleTime=-1
  Transfer Fcn2 : TransferFcn  Numerator=2500  Denominator=conv([1 50], [1 50])
  ReferencePosition : Outport
  ReferenceSpeed : Outport  Port=2
  wires:
  Transfer Fcn2/1 -> Integrator/1, To Workspace1/1, ReferenceSpeed/1
  Prepocessor Elevation/3(PositionRef) -> Terminator1/1
  Integrator/1 -> To Workspace/1, ReferencePosition/1
  Prepocessor Elevation/1(deltaP) -> Terminator/1
  Prepocessor Elevation/2(speed) -> Transfer Fcn2/1
  Astrometry Computation/1 -> Prepocessor Elevation/1(El)

== system Telescope_model_MPC/Telescope Model/Azimuth Model/Noise Model/None Noise ==
  Clock : Clock
  Constant : Constant  Value=0
  Constant3 : Constant  Value=0
  Divide : Product  Inputs=**
  Divide1 : Product  Inputs=**
  d_out : Outport
  d_in : Outport  Port=2
  wires:
  Constant3/1 -> Divide/2
  Constant/1 -> Divide1/1
  Clock/1 -> Divide/1, Divide1/2
  Divide1/1 -> d_out/1
  Divide/1 -> d_in/1

== system Telescope_model_MPC/Telescope Model/Azimuth Model/Noise Model/Von Karman Torque PSD ==
  Add : Sum  Inputs=+
  Add2 : Sum
  Clock2 : Clock
  Constant : Constant  Value=0
  Constant1 : Constant  Value=4/VonKarman.v_mean^2
  Constant2 : Constant  Value=100
  Constant3 : Constant  Value=VonKarman.f
  Constant4 : Constant  Value=VonKarman.phi
  Cos1 : Trigonometry  Operator=cos
  Divide{1..6} (6 alike) : Product  Inputs=**
  Gain : Gain  Gain=VonKarman.alpha
  Gain1 : Gain  Gain=2*VonKarman.df
  Gain2 : Gain  Gain=2*pi
  Sqrt : Sqrt
  Square : Math  Operator=square
  Square1 : Math  Operator=square
  Step : Step  SampleTime=0
  Sv : Subsystem
  Transfer Fcn : TransferFcn  Numerator=[100]  Denominator=conv([1 10], [1 10])
  X : Subsystem
  d_out : Outport
  d_in : Outport  Port=2
  wires:
  Divide1/1 -> Transfer Fcn/1
  Cos1/1 -> Divide3/1
  Step/1 -> Divide1/2
  Divide4/1 -> Add2/1
  Gain1/1 -> Sqrt/1
  X/1(Out_X) -> Square/1
  Sqrt/1 -> Divide5/1
  Gain2/1 -> Divide4/2
  Clock2/1 -> Divide4/1
  Sv/1(Out_Sv) -> Divide2/2
  Constant2/1 -> Square1/1
  Add2/1 -> Cos1/1
  Divide2/1 -> Gain1/1
  Divide3/1 -> Add/1
  Square/1 -> Divide2/1
  Add/1 -> Divide1/1
  Constant1/1 -> Divide6/1
  Constant3/1 -> X/1(f), Sv/1(f), Gain2/1
  Divide5/1 -> Divide3/2
  Constant4/1 -> Add2/2
  Square1/1 -> Divide6/2
  Divide6/1 -> Divide5/2
  Transfer Fcn/1 -> Gain/1
  Constant/1 -> d_out/1
  Gain/1 -> d_in/1

== system Telescope_model_MPC/Telescope Model/Azimuth Model/Noise Model/White Noise Output ==
  Band-Limited White Noise : simulink/Sources/Band-Limited White Noise  Cov=[0.04]  Ts=0.02  seed=[23341]
  Band-Limited White Noise1 : simulink/Sources/Band-Limited White Noise  Cov=400000  Ts=0.02  seed=[23341]
  Constant1 : Constant  Value=0
  Gain : Gain  Gain=Deg2Arcs
  Scope : Scope  NumInputPorts=3
  d_out : Outport
  d_in : Outport  Port=2
  wires:
  Band-Limited White Noise/1 -> Scope/1, Gain/1
  Band-Limited White Noise1/1 -> Scope/2
  Gain/1 -> Scope/3, d_out/1
  Constant1/1 -> d_in/1

== system Telescope_model_MPC/Telescope Model/Elevation Model/Noise Model/None Noise ==
  Clock : Clock
  Constant : Constant  Value=0
  Constant3 : Constant  Value=0
  Divide : Product  Inputs=**
  Divide1 : Product  Inputs=**
  d_out : Outport
  d_in : Outport  Port=2
  wires:
  Constant3/1 -> Divide/2
  Constant/1 -> Divide1/1
  Clock/1 -> Divide/1, Divide1/2
  Divide1/1 -> d_out/1
  Divide/1 -> d_in/1

== system Telescope_model_MPC/Telescope Model/Elevation Model/Noise Model/Von Karman Torque PSD ==
  Add : Sum  Inputs=+
  Add2 : Sum
  Clock2 : Clock
  Constant : Constant  Value=0
  Constant1 : Constant  Value=4/VonKarman.v_mean^2
  Constant2 : Constant  Value=100
  Constant3 : Constant  Value=VonKarman.f
  Constant4 : Constant  Value=VonKarman.phi
  Cos1 : Trigonometry  Operator=cos
  Divide{1..6} (6 alike) : Product  Inputs=**
  Gain : Gain  Gain=VonKarman.alpha
  Gain1 : Gain  Gain=2*VonKarman.df
  Gain2 : Gain  Gain=2*pi
  Sqrt : Sqrt
  Square : Math  Operator=square
  Square1 : Math  Operator=square
  Step : Step  SampleTime=0
  Sv : Subsystem
  Transfer Fcn : TransferFcn  Numerator=[100]  Denominator=conv([1 10], [1 10])
  X : Subsystem
  d_out : Outport
  d_in : Outport  Port=2
  wires:
  Divide1/1 -> Transfer Fcn/1
  Cos1/1 -> Divide3/1
  Step/1 -> Divide1/2
  Divide4/1 -> Add2/1
  Gain1/1 -> Sqrt/1
  X/1(Out_X) -> Square/1
  Sqrt/1 -> Divide5/1
  Gain2/1 -> Divide4/2
  Clock2/1 -> Divide4/1
  Sv/1(Out_Sv) -> Divide2/2
  Constant2/1 -> Square1/1
  Add2/1 -> Cos1/1
  Divide2/1 -> Gain1/1
  Divide3/1 -> Add/1
  Square/1 -> Divide2/1
  Add/1 -> Divide1/1
  Constant1/1 -> Divide6/1
  Constant3/1 -> X/1(f), Sv/1(f), Gain2/1
  Divide5/1 -> Divide3/2
  Constant4/1 -> Add2/2
  Square1/1 -> Divide6/2
  Divide6/1 -> Divide5/2
  Transfer Fcn/1 -> Gain/1
  Constant/1 -> d_out/1
  Gain/1 -> d_in/1

== system Telescope_model_MPC/Telescope Model/Elevation Model/Noise Model/White Noise Output ==
  Band-Limited White Noise : simulink/Sources/Band-Limited White Noise  Cov=[0.04]  Ts=0.02  seed=[23341]
  Band-Limited White Noise1 : simulink/Sources/Band-Limited White Noise  Cov=400000  Ts=0.02  seed=[23341]
  Constant1 : Constant  Value=0
  Gain : Gain  Gain=Deg2Arcs
  Scope : Scope  NumInputPorts=3
  d_out : Outport
  d_in : Outport  Port=2
  wires:
  Band-Limited White Noise/1 -> Scope/1, Gain/1
  Band-Limited White Noise1/1 -> Scope/2
  Gain/1 -> Scope/3, d_out/1
  Constant1/1 -> d_in/1

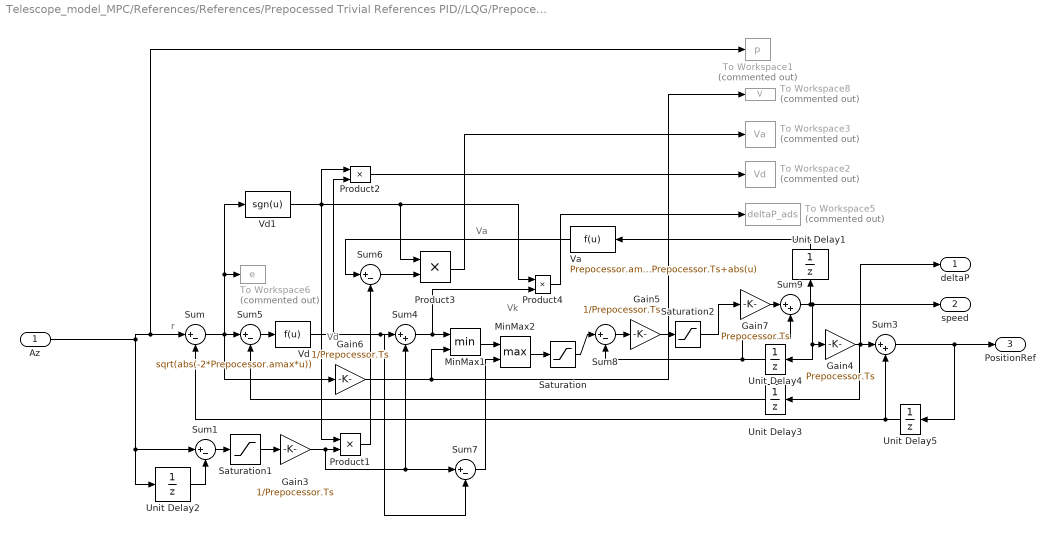
== system Telescope_model_MPC/References/References/Prepocessed Trivial References PID//LQG/Prepocessor Azimuth/Prepocessor Elevation ==
  note: Vd
  note: Va
  note: Vk
  note: r
  Az : Inport
  Gain3 : Gain  Gain=1/Prepocessor.Ts
  Gain4 : Gain  Gain=Prepocessor.Ts
  Gain5 : Gain  Gain=1/Prepocessor.Ts
  Gain6 : Gain  Gain=1/Prepocessor.Ts
  Gain7 : Gain  Gain=Prepocessor.Ts
  MinMax1 : MinMax  Inputs=2
  MinMax2 : MinMax  Function=max  Inputs=2
  Product{1..4} (4 alike) : Product
  Saturation : Saturate  UpperLimit=Prepocessor.vmax  LowerLimit=-Prepocessor.vmax
  Saturation1 : Saturate  UpperLimit=Prepocessor.vmax*Prepocessor.Ts  LowerLimit=-Prepocessor.vmax*Prepocessor.Ts
  Saturation2 : Saturate  UpperLimit=Prepocessor.amax  LowerLimit=-Prepocessor.amax
  Sum{,1,5..8} (6 alike) : Sum  Inputs=|+-
  Sum3 : Sum  Inputs=|++
  Sum4 : Sum  Inputs=|++
  Sum9 : Sum  Inputs=|++
  To Workspace1 : ToWorkspace  Commented=on  VariableName=p  SampleTime=-1
  To Workspace2 : ToWorkspace  Commented=on  VariableName=Vd  SampleTime=-1
  To Workspace3 : ToWorkspace  Commented=on  VariableName=Va  SampleTime=-1
  To Workspace5 : ToWorkspace  Commented=on  VariableName=deltaP_ads  SampleTime=-1
  To Workspace6 : ToWorkspace  Commented=on  VariableName=e  SampleTime=-1
  To Workspace8 : ToWorkspace  Commented=on  VariableName=V  SampleTime=-1
  Unit Delay{1..4} (4 alike) : UnitDelay  SampleTime=-1  HasFrameUpgradeWarning=on
  Unit Delay5 : UnitDelay  InitialCondition=Prepocessor.p0az  SampleTime=-1  HasFrameUpgradeWarning=on
  Va : Fcn  Expr=Prepocessor.amax*Prepocessor.Ts+abs(u)
  Vd : Fcn  Expr=sqrt(abs(-2*Prepocessor.amax*u))
  Vd1 : Fcn  Expr=sgn(u)
  deltaP : Outport
  speed : Outport  Port=2
  PositionRef : Outport  Port=3
  wires:
  Unit Delay5/1 -> Sum/2, Sum3/2
  Product4/1 -> To Workspace5/1
  Az/1 -> Unit Delay2/1, Sum1/1, Sum/1, To Workspace1/1
  Product2/1 -> To Workspace2/1
  Product3/1 -> To Workspace3/1
  Vd/1 -> Product2/2, Sum7/2, Sum4/1
  Sum4/1 -> Product4/2, MinMax1/1
  Unit Delay3/1 -> Sum5/2
  Product1/1 -> Sum6/2
  Gain4/1 -> deltaP/1, Sum3/1, Unit Delay3/1
  Vd1/1 -> Product2/1, Product1/1, Product4/1, Product3/1
  Saturation2/1 -> Gain7/1
  Sum7/1 -> MinMax2/2
  Va/1 -> Sum6/1
  Sum1/1 -> Saturation1/1
  Sum/1 -> Sum5/1, Gain6/1, Vd1/1, To Workspace6/1
  Unit Delay2/1 -> Sum1/2
  Gain7/1 -> Sum9/1
  Sum9/1 -> speed/1, Unit Delay4/1, Gain4/1, Unit Delay1/1
  Unit Delay4/1 -> Sum8/2, Sum9/2
  Gain6/1 -> MinMax1/2, To Workspace8/1
  MinMax1/1 -> MinMax2/1
  Gain3/1 -> Sum7/1, Sum4/2, Product1/2
  Sum6/1 -> Product3/2
  Saturation1/1 -> Gain3/1
  Saturation/1 -> Sum8/1
  Sum8/1 -> Gain5/1
  Sum5/1 -> Vd/1
  MinMax2/1 -> Saturation/1
  Unit Delay1/1 -> Va/1
  Gain5/1 -> Saturation2/1
  Sum3/1 -> Unit Delay5/1, PositionRef/1

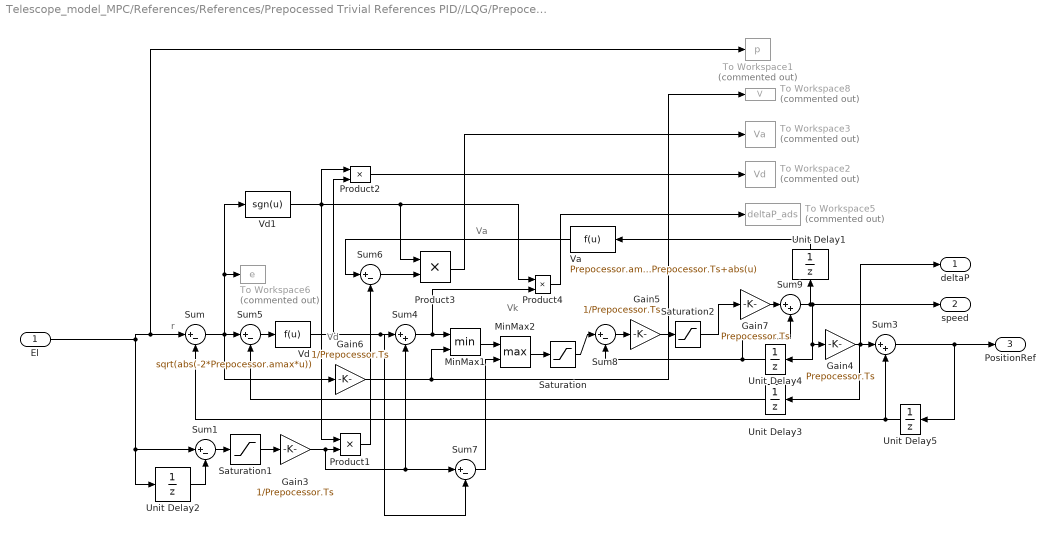
== system Telescope_model_MPC/References/References/Prepocessed Trivial References PID//LQG/Prepocessor Elavation/Prepocessor Elevation ==
  note: Vd
  note: Va
  note: Vk
  note: r
  El : Inport
  Gain3 : Gain  Gain=1/Prepocessor.Ts
  Gain4 : Gain  Gain=Prepocessor.Ts
  Gain5 : Gain  Gain=1/Prepocessor.Ts
  Gain6 : Gain  Gain=1/Prepocessor.Ts
  Gain7 : Gain  Gain=Prepocessor.Ts
  MinMax1 : MinMax  Inputs=2
  MinMax2 : MinMax  Function=max  Inputs=2
  Product{1..4} (4 alike) : Product
  Saturation : Saturate  UpperLimit=Prepocessor.vmax  LowerLimit=-Prepocessor.vmax
  Saturation1 : Saturate  UpperLimit=Prepocessor.vmax*Prepocessor.Ts  LowerLimit=-Prepocessor.vmax*Prepocessor.Ts
  Saturation2 : Saturate  UpperLimit=Prepocessor.amax  LowerLimit=-Prepocessor.amax
  Sum{,1,5..8} (6 alike) : Sum  Inputs=|+-
  Sum3 : Sum  Inputs=|++
  Sum4 : Sum  Inputs=|++
  Sum9 : Sum  Inputs=|++
  To Workspace1 : ToWorkspace  Commented=on  VariableName=p  SampleTime=-1
  To Workspace2 : ToWorkspace  Commented=on  VariableName=Vd  SampleTime=-1
  To Workspace3 : ToWorkspace  Commented=on  VariableName=Va  SampleTime=-1
  To Workspace5 : ToWorkspace  Commented=on  VariableName=deltaP_ads  SampleTime=-1
  To Workspace6 : ToWorkspace  Commented=on  VariableName=e  SampleTime=-1
  To Workspace8 : ToWorkspace  Commented=on  VariableName=V  SampleTime=-1
  Unit Delay{1..4} (4 alike) : UnitDelay  SampleTime=-1  HasFrameUpgradeWarning=on
  Unit Delay5 : UnitDelay  InitialCondition=Prepocessor.p0el  SampleTime=-1  HasFrameUpgradeWarning=on
  Va : Fcn  Expr=Prepocessor.amax*Prepocessor.Ts+abs(u)
  Vd : Fcn  Expr=sqrt(abs(-2*Prepocessor.amax*u))
  Vd1 : Fcn  Expr=sgn(u)
  deltaP : Outport
  speed : Outport  Port=2
  PositionRef : Outport  Port=3
  wires:
  Unit Delay5/1 -> Sum/2, Sum3/2
  Product4/1 -> To Workspace5/1
  El/1 -> Unit Delay2/1, Sum1/1, Sum/1, To Workspace1/1
  Product2/1 -> To Workspace2/1
  Product3/1 -> To Workspace3/1
  Vd/1 -> Product2/2, Sum7/2, Sum4/1
  Sum4/1 -> Product4/2, MinMax1/1
  Unit Delay3/1 -> Sum5/2
  Product1/1 -> Sum6/2
  Gain4/1 -> deltaP/1, Sum3/1, Unit Delay3/1
  Vd1/1 -> Product2/1, Product1/1, Product4/1, Product3/1
  Saturation2/1 -> Gain7/1
  Sum7/1 -> MinMax2/2
  Va/1 -> Sum6/1
  Sum1/1 -> Saturation1/1
  Sum/1 -> Sum5/1, Gain6/1, Vd1/1, To Workspace6/1
  Unit Delay2/1 -> Sum1/2
  Gain7/1 -> Sum9/1
  Sum9/1 -> speed/1, Unit Delay4/1, Gain4/1, Unit Delay1/1
  Unit Delay4/1 -> Sum8/2, Sum9/2
  Gain6/1 -> MinMax1/2, To Workspace8/1
  MinMax1/1 -> MinMax2/1
  Gain3/1 -> Sum7/1, Sum4/2, Product1/2
  Sum6/1 -> Product3/2
  Saturation1/1 -> Gain3/1
  Saturation/1 -> Sum8/1
  Sum8/1 -> Gain5/1
  Sum5/1 -> Vd/1
  MinMax2/1 -> Saturation/1
  Unit Delay1/1 -> Va/1
  Gain5/1 -> Saturation2/1
  Sum3/1 -> Unit Delay5/1, PositionRef/1

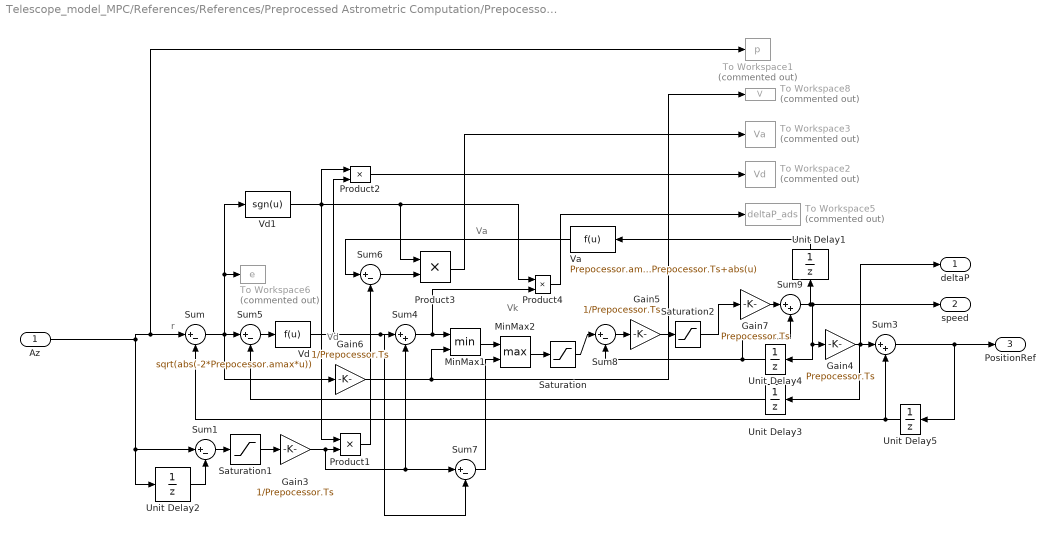
== system Telescope_model_MPC/References/References/Preprocessed Astrometric Computation/Prepocessor Azimuth/Prepocessor Elevation ==
  note: Vd
  note: Va
  note: Vk
  note: r
  Az : Inport
  Gain3 : Gain  Gain=1/Prepocessor.Ts
  Gain4 : Gain  Gain=Prepocessor.Ts
  Gain5 : Gain  Gain=1/Prepocessor.Ts
  Gain6 : Gain  Gain=1/Prepocessor.Ts
  Gain7 : Gain  Gain=Prepocessor.Ts
  MinMax1 : MinMax  Inputs=2
  MinMax2 : MinMax  Function=max  Inputs=2
  Product{1..4} (4 alike) : Product
  Saturation : Saturate  UpperLimit=Prepocessor.vmax  LowerLimit=-Prepocessor.vmax
  Saturation1 : Saturate  UpperLimit=Prepocessor.vmax*Prepocessor.Ts  LowerLimit=-Prepocessor.vmax*Prepocessor.Ts
  Saturation2 : Saturate  UpperLimit=Prepocessor.amax  LowerLimit=-Prepocessor.amax
  Sum{,1,5..8} (6 alike) : Sum  Inputs=|+-
  Sum3 : Sum  Inputs=|++
  Sum4 : Sum  Inputs=|++
  Sum9 : Sum  Inputs=|++
  To Workspace1 : ToWorkspace  Commented=on  VariableName=p  SampleTime=-1
  To Workspace2 : ToWorkspace  Commented=on  VariableName=Vd  SampleTime=-1
  To Workspace3 : ToWorkspace  Commented=on  VariableName=Va  SampleTime=-1
  To Workspace5 : ToWorkspace  Commented=on  VariableName=deltaP_ads  SampleTime=-1
  To Workspace6 : ToWorkspace  Commented=on  VariableName=e  SampleTime=-1
  To Workspace8 : ToWorkspace  Commented=on  VariableName=V  SampleTime=-1
  Unit Delay{1..4} (4 alike) : UnitDelay  SampleTime=-1  HasFrameUpgradeWarning=on
  Unit Delay5 : UnitDelay  InitialCondition=Prepocessor.p0az  SampleTime=-1  HasFrameUpgradeWarning=on
  Va : Fcn  Expr=Prepocessor.amax*Prepocessor.Ts+abs(u)
  Vd : Fcn  Expr=sqrt(abs(-2*Prepocessor.amax*u))
  Vd1 : Fcn  Expr=sgn(u)
  deltaP : Outport
  speed : Outport  Port=2
  PositionRef : Outport  Port=3
  wires:
  Unit Delay5/1 -> Sum/2, Sum3/2
  Product4/1 -> To Workspace5/1
  Az/1 -> Unit Delay2/1, Sum1/1, Sum/1, To Workspace1/1
  Product2/1 -> To Workspace2/1
  Product3/1 -> To Workspace3/1
  Vd/1 -> Product2/2, Sum7/2, Sum4/1
  Sum4/1 -> Product4/2, MinMax1/1
  Unit Delay3/1 -> Sum5/2
  Product1/1 -> Sum6/2
  Gain4/1 -> deltaP/1, Sum3/1, Unit Delay3/1
  Vd1/1 -> Product2/1, Product1/1, Product4/1, Product3/1
  Saturation2/1 -> Gain7/1
  Sum7/1 -> MinMax2/2
  Va/1 -> Sum6/1
  Sum1/1 -> Saturation1/1
  Sum/1 -> Sum5/1, Gain6/1, Vd1/1, To Workspace6/1
  Unit Delay2/1 -> Sum1/2
  Gain7/1 -> Sum9/1
  Sum9/1 -> speed/1, Unit Delay4/1, Gain4/1, Unit Delay1/1
  Unit Delay4/1 -> Sum8/2, Sum9/2
  Gain6/1 -> MinMax1/2, To Workspace8/1
  MinMax1/1 -> MinMax2/1
  Gain3/1 -> Sum7/1, Sum4/2, Product1/2
  Sum6/1 -> Product3/2
  Saturation1/1 -> Gain3/1
  Saturation/1 -> Sum8/1
  Sum8/1 -> Gain5/1
  Sum5/1 -> Vd/1
  MinMax2/1 -> Saturation/1
  Unit Delay1/1 -> Va/1
  Gain5/1 -> Saturation2/1
  Sum3/1 -> Unit Delay5/1, PositionRef/1
